simulink model "aa_IOT"  (R2024b)
settings: Solver=VariableStepAuto  StartTime=0.0  StopTime=0.05  RelTol=1e-3
undefined symbols (not defined in the file): Acid, Ion, Lead, Lithium, sigbuilder_block
libraries: spsBreakerLib x120, spsBatteryLib x82, spsSeriesRLCBranchLib x74, spsIdealSwitchLib x37, spsVoltageMeasurementLib x29, slpidlib x17, spsMosfetLib x17, spsPWMGeneratorDCDCLib x11, spsDiodeLib x10, spsIGBTLib x4, spsCurrentMeasurementLib x4, spsThreePhaseSeriesRLCLoadLib x2
(part 3 of 6)

== system aa_IOT/Subsystem11/Subsystem29 ==
  Battery : spsBatteryLib/Battery  BatType=Lithium-Ion  NomV=12  NomQ=10  SOC=95  Batt_Tr=30  PresetModel=on  MaxQ=10  MinV=9  FullV=13.9678  Dis_rate=4.3478  R=0.012  Normal_OP=9.0435  expZone="[12.9646     0.491304]"
  Breaker{,1..3} (4 alike) : spsBreakerLib/Breaker  InitialState=0  SwitchingTimes="[1/60  5/60]"  External=on  BreakerResistance=0.01  SnubberResistance=1e6  SnubberCapacitance=inf  Measurements=None  MoreParameters=on  NoBreakLoop=off
  Bus Selector : BusSelector  OutputSignals=SOC (%),Current (A),Voltage (V)
  Scope : Scope  NumInputPorts=3
  Series RLC Branch : spsSeriesRLCBranchLib/Series RLC Branch  LConnTagsString=__new0  RConnTagsString=__new0  BranchType=R  Resistance=1  Inductance=1e-3  SetiL0=off  InitialCurrent=0  Capacitance=1e-6  Setx0=off  InitialVoltage=0  Measurements=None
  + : PMIOPort  Side=Right
  - : PMIOPort  Port=2  Side=Right
  tag scope: s22=global
  wires:
  Battery/1 -> Bus Selector/1
  [c22] -> Breaker3/1, Breaker/1
  Bus Selector/2 -> Scope/2  "<Current (A)>"
  [d22] -> Breaker1/1, Breaker2/1
  Bus Selector/3 -> Scope/3  "<Voltage (V)>"
  Bus Selector/1 -> [s22], Scope/1  "<SOC (%)>"
  connections:
  Breaker2/LConn1 -- Breaker3/RConn1 -- Battery/LConn2
  Breaker1/LConn1 -- Battery/LConn1 -- Breaker/RConn1
  +/RConn1 -- Breaker/LConn1
  Series RLC Branch/LConn1 -- Breaker2/RConn1
  Series RLC Branch/RConn1 -- Breaker1/RConn1
  -/RConn1 -- Breaker3/LConn1

== system aa_IOT/Subsystem11/Subsystem3 ==
  Battery : spsBatteryLib/Battery  BatType=Lithium-Ion  NomV=12  NomQ=10  SOC=95  Batt_Tr=30  PresetModel=on  MaxQ=10  MinV=9  FullV=13.9678  Dis_rate=4.3478  R=0.012  Normal_OP=9.0435  expZone="[12.9646     0.491304]"
  Breaker{,1..3} (4 alike) : spsBreakerLib/Breaker  InitialState=0  SwitchingTimes="[1/60  5/60]"  External=on  BreakerResistance=0.01  SnubberResistance=1e6  SnubberCapacitance=inf  Measurements=None  MoreParameters=on  NoBreakLoop=off
  Bus Selector : BusSelector  OutputSignals=SOC (%),Current (A),Voltage (V)
  Scope : Scope  NumInputPorts=3
  Series RLC Branch : spsSeriesRLCBranchLib/Series RLC Branch  LConnTagsString=__new0  RConnTagsString=__new0  BranchType=R  Resistance=1  Inductance=1e-3  SetiL0=off  InitialCurrent=0  Capacitance=1e-6  Setx0=off  InitialVoltage=0  Measurements=None
  + : PMIOPort  Side=Right
  - : PMIOPort  Port=2  Side=Right
  tag scope: s4=global
  wires:
  Battery/1 -> Bus Selector/1
  [c4] -> Breaker3/1, Breaker/1
  Bus Selector/2 -> Scope/2  "<Current (A)>"
  [d4] -> Breaker1/1, Breaker2/1
  Bus Selector/3 -> Scope/3  "<Voltage (V)>"
  Bus Selector/1 -> [s4], Scope/1  "<SOC (%)>"
  connections:
  Breaker2/LConn1 -- Breaker3/RConn1 -- Battery/LConn2
  Breaker1/LConn1 -- Battery/LConn1 -- Breaker/RConn1
  +/RConn1 -- Breaker/LConn1
  Series RLC Branch/LConn1 -- Breaker2/RConn1
  Series RLC Branch/RConn1 -- Breaker1/RConn1
  -/RConn1 -- Breaker3/LConn1

== system aa_IOT/Subsystem11/Subsystem4 ==
  Battery : spsBatteryLib/Battery  BatType=Lithium-Ion  NomV=12  NomQ=10  SOC=95  Batt_Tr=30  PresetModel=on  MaxQ=10  MinV=9  FullV=13.9678  Dis_rate=4.3478  R=0.012  Normal_OP=9.0435  expZone="[12.9646     0.491304]"
  Breaker{,1..3} (4 alike) : spsBreakerLib/Breaker  InitialState=0  SwitchingTimes="[1/60  5/60]"  External=on  BreakerResistance=0.01  SnubberResistance=1e6  SnubberCapacitance=inf  Measurements=None  MoreParameters=on  NoBreakLoop=off
  Bus Selector : BusSelector  OutputSignals=SOC (%),Current (A),Voltage (V)
  Scope : Scope  NumInputPorts=3
  Series RLC Branch : spsSeriesRLCBranchLib/Series RLC Branch  LConnTagsString=__new0  RConnTagsString=__new0  BranchType=R  Resistance=1  Inductance=1e-3  SetiL0=off  InitialCurrent=0  Capacitance=1e-6  Setx0=off  InitialVoltage=0  Measurements=None
  + : PMIOPort  Side=Right
  - : PMIOPort  Port=2  Side=Right
  tag scope: s3=global
  wires:
  Battery/1 -> Bus Selector/1
  [c3] -> Breaker3/1, Breaker/1
  Bus Selector/2 -> Scope/2  "<Current (A)>"
  [d3] -> Breaker1/1, Breaker2/1
  Bus Selector/3 -> Scope/3  "<Voltage (V)>"
  Bus Selector/1 -> [s3], Scope/1  "<SOC (%)>"
  connections:
  Breaker2/LConn1 -- Breaker3/RConn1 -- Battery/LConn2
  Breaker1/LConn1 -- Battery/LConn1 -- Breaker/RConn1
  +/RConn1 -- Breaker/LConn1
  Series RLC Branch/LConn1 -- Breaker2/RConn1
  Series RLC Branch/RConn1 -- Breaker1/RConn1
  -/RConn1 -- Breaker3/LConn1

== system aa_IOT/Subsystem11/Subsystem5 ==
  Battery : spsBatteryLib/Battery  BatType=Lithium-Ion  NomV=12  NomQ=10  SOC=95  Batt_Tr=30  PresetModel=on  MaxQ=10  MinV=9  FullV=13.9678  Dis_rate=4.3478  R=0.012  Normal_OP=9.0435  expZone="[12.9646     0.491304]"
  Breaker{,1..3} (4 alike) : spsBreakerLib/Breaker  InitialState=0  SwitchingTimes="[1/60  5/60]"  External=on  BreakerResistance=0.01  SnubberResistance=1e6  SnubberCapacitance=inf  Measurements=None  MoreParameters=on  NoBreakLoop=off
  Bus Selector : BusSelector  OutputSignals=SOC (%),Current (A),Voltage (V)
  Scope : Scope  NumInputPorts=3
  Series RLC Branch : spsSeriesRLCBranchLib/Series RLC Branch  LConnTagsString=__new0  RConnTagsString=__new0  BranchType=R  Resistance=1  Inductance=1e-3  SetiL0=off  InitialCurrent=0  Capacitance=1e-6  Setx0=off  InitialVoltage=0  Measurements=None
  + : PMIOPort  Side=Right
  - : PMIOPort  Port=2  Side=Right
  tag scope: s2=global
  wires:
  Battery/1 -> Bus Selector/1
  [c2] -> Breaker3/1, Breaker/1
  Bus Selector/2 -> Scope/2  "<Current (A)>"
  [d2] -> Breaker1/1, Breaker2/1
  Bus Selector/3 -> Scope/3  "<Voltage (V)>"
  Bus Selector/1 -> [s2], Scope/1  "<SOC (%)>"
  connections:
  Breaker2/LConn1 -- Breaker3/RConn1 -- Battery/LConn2
  Breaker1/LConn1 -- Battery/LConn1 -- Breaker/RConn1
  +/RConn1 -- Breaker/LConn1
  Series RLC Branch/LConn1 -- Breaker2/RConn1
  Series RLC Branch/RConn1 -- Breaker1/RConn1
  -/RConn1 -- Breaker3/LConn1

== system aa_IOT/Subsystem11/Subsystem6 ==
  Battery : spsBatteryLib/Battery  BatType=Lithium-Ion  NomV=12  NomQ=10  SOC=95  Batt_Tr=30  PresetModel=on  MaxQ=10  MinV=9  FullV=13.9678  Dis_rate=4.3478  R=0.012  Normal_OP=9.0435  expZone="[12.9646     0.491304]"
  Breaker{,1..3} (4 alike) : spsBreakerLib/Breaker  InitialState=0  SwitchingTimes="[1/60  5/60]"  External=on  BreakerResistance=0.01  SnubberResistance=1e6  SnubberCapacitance=inf  Measurements=None  MoreParameters=on  NoBreakLoop=off
  Bus Selector : BusSelector  OutputSignals=SOC (%),Current (A),Voltage (V)
  Scope : Scope  NumInputPorts=3
  Series RLC Branch : spsSeriesRLCBranchLib/Series RLC Branch  LConnTagsString=__new0  RConnTagsString=__new0  BranchType=R  Resistance=1  Inductance=1e-3  SetiL0=off  InitialCurrent=0  Capacitance=1e-6  Setx0=off  InitialVoltage=0  Measurements=None
  + : PMIOPort  Side=Right
  - : PMIOPort  Port=2  Side=Right
  tag scope: s15=global
  wires:
  Battery/1 -> Bus Selector/1
  [c15] -> Breaker3/1, Breaker/1
  Bus Selector/2 -> Scope/2  "<Current (A)>"
  [d15] -> Breaker1/1, Breaker2/1
  Bus Selector/3 -> Scope/3  "<Voltage (V)>"
  Bus Selector/1 -> [s15], Scope/1  "<SOC (%)>"
  connections:
  Breaker2/LConn1 -- Breaker3/RConn1 -- Battery/LConn2
  Breaker1/LConn1 -- Battery/LConn1 -- Breaker/RConn1
  +/RConn1 -- Breaker/LConn1
  Series RLC Branch/LConn1 -- Breaker2/RConn1
  Series RLC Branch/RConn1 -- Breaker1/RConn1
  -/RConn1 -- Breaker3/LConn1

== system aa_IOT/Subsystem11/Subsystem7 ==
  Battery : spsBatteryLib/Battery  BatType=Lithium-Ion  NomV=12  NomQ=10  SOC=95  Batt_Tr=30  PresetModel=on  MaxQ=10  MinV=9  FullV=13.9678  Dis_rate=4.3478  R=0.012  Normal_OP=9.0435  expZone="[12.9646     0.491304]"
  Breaker{,1..3} (4 alike) : spsBreakerLib/Breaker  InitialState=0  SwitchingTimes="[1/60  5/60]"  External=on  BreakerResistance=0.01  SnubberResistance=1e6  SnubberCapacitance=inf  Measurements=None  MoreParameters=on  NoBreakLoop=off
  Bus Selector : BusSelector  OutputSignals=SOC (%),Current (A),Voltage (V)
  Scope : Scope  NumInputPorts=3
  Series RLC Branch : spsSeriesRLCBranchLib/Series RLC Branch  LConnTagsString=__new0  RConnTagsString=__new0  BranchType=R  Resistance=1  Inductance=1e-3  SetiL0=off  InitialCurrent=0  Capacitance=1e-6  Setx0=off  InitialVoltage=0  Measurements=None
  + : PMIOPort  Side=Right
  - : PMIOPort  Port=2  Side=Right
  tag scope: s11=global
  wires:
  Battery/1 -> Bus Selector/1
  [c11] -> Breaker3/1, Breaker/1
  Bus Selector/2 -> Scope/2  "<Current (A)>"
  [d11] -> Breaker1/1, Breaker2/1
  Bus Selector/3 -> Scope/3  "<Voltage (V)>"
  Bus Selector/1 -> [s11], Scope/1  "<SOC (%)>"
  connections:
  Breaker2/LConn1 -- Breaker3/RConn1 -- Battery/LConn2
  Breaker1/LConn1 -- Battery/LConn1 -- Breaker/RConn1
  +/RConn1 -- Breaker/LConn1
  Series RLC Branch/LConn1 -- Breaker2/RConn1
  Series RLC Branch/RConn1 -- Breaker1/RConn1
  -/RConn1 -- Breaker3/LConn1

== system aa_IOT/Subsystem11/Subsystem8 ==
  Battery : spsBatteryLib/Battery  BatType=Lithium-Ion  NomV=12  NomQ=10  SOC=95  Batt_Tr=30  PresetModel=on  MaxQ=10  MinV=9  FullV=13.9678  Dis_rate=4.3478  R=0.012  Normal_OP=9.0435  expZone="[12.9646     0.491304]"
  Breaker{,1..3} (4 alike) : spsBreakerLib/Breaker  InitialState=0  SwitchingTimes="[1/60  5/60]"  External=on  BreakerResistance=0.01  SnubberResistance=1e6  SnubberCapacitance=inf  Measurements=None  MoreParameters=on  NoBreakLoop=off
  Bus Selector : BusSelector  OutputSignals=SOC (%),Current (A),Voltage (V)
  Scope : Scope  NumInputPorts=3
  Series RLC Branch : spsSeriesRLCBranchLib/Series RLC Branch  LConnTagsString=__new0  RConnTagsString=__new0  BranchType=R  Resistance=1  Inductance=1e-3  SetiL0=off  InitialCurrent=0  Capacitance=1e-6  Setx0=off  InitialVoltage=0  Measurements=None
  + : PMIOPort  Side=Right
  - : PMIOPort  Port=2  Side=Right
  tag scope: s19=global
  wires:
  Battery/1 -> Bus Selector/1
  [c19] -> Breaker3/1, Breaker/1
  Bus Selector/2 -> Scope/2  "<Current (A)>"
  [d19] -> Breaker1/1, Breaker2/1
  Bus Selector/3 -> Scope/3  "<Voltage (V)>"
  Bus Selector/1 -> [s19], Scope/1  "<SOC (%)>"
  connections:
  Breaker2/LConn1 -- Breaker3/RConn1 -- Battery/LConn2
  Breaker1/LConn1 -- Battery/LConn1 -- Breaker/RConn1
  +/RConn1 -- Breaker/LConn1
  Series RLC Branch/LConn1 -- Breaker2/RConn1
  Series RLC Branch/RConn1 -- Breaker1/RConn1
  -/RConn1 -- Breaker3/LConn1

== system aa_IOT/Subsystem11/Subsystem9 ==
  Battery : spsBatteryLib/Battery  BatType=Lithium-Ion  NomV=12  NomQ=10  SOC=95  Batt_Tr=30  PresetModel=on  MaxQ=10  MinV=9  FullV=13.9678  Dis_rate=4.3478  R=0.012  Normal_OP=9.0435  expZone="[12.9646     0.491304]"
  Breaker{,1..3} (4 alike) : spsBreakerLib/Breaker  InitialState=0  SwitchingTimes="[1/60  5/60]"  External=on  BreakerResistance=0.01  SnubberResistance=1e6  SnubberCapacitance=inf  Measurements=None  MoreParameters=on  NoBreakLoop=off
  Bus Selector : BusSelector  OutputSignals=SOC (%),Current (A),Voltage (V)
  Scope : Scope  NumInputPorts=3
  Series RLC Branch : spsSeriesRLCBranchLib/Series RLC Branch  LConnTagsString=__new0  RConnTagsString=__new0  BranchType=R  Resistance=1  Inductance=1e-3  SetiL0=off  InitialCurrent=0  Capacitance=1e-6  Setx0=off  InitialVoltage=0  Measurements=None
  + : PMIOPort  Side=Right
  - : PMIOPort  Port=2  Side=Right
  tag scope: s20=global
  wires:
  Battery/1 -> Bus Selector/1
  [c20] -> Breaker3/1, Breaker/1
  Bus Selector/2 -> Scope/2  "<Current (A)>"
  [d20] -> Breaker1/1, Breaker2/1
  Bus Selector/3 -> Scope/3  "<Voltage (V)>"
  Bus Selector/1 -> [s20], Scope/1  "<SOC (%)>"
  connections:
  Breaker2/LConn1 -- Breaker3/RConn1 -- Battery/LConn2
  Breaker1/LConn1 -- Battery/LConn1 -- Breaker/RConn1
  +/RConn1 -- Breaker/LConn1
  Series RLC Branch/LConn1 -- Breaker2/RConn1
  Series RLC Branch/RConn1 -- Breaker1/RConn1
  -/RConn1 -- Breaker3/LConn1

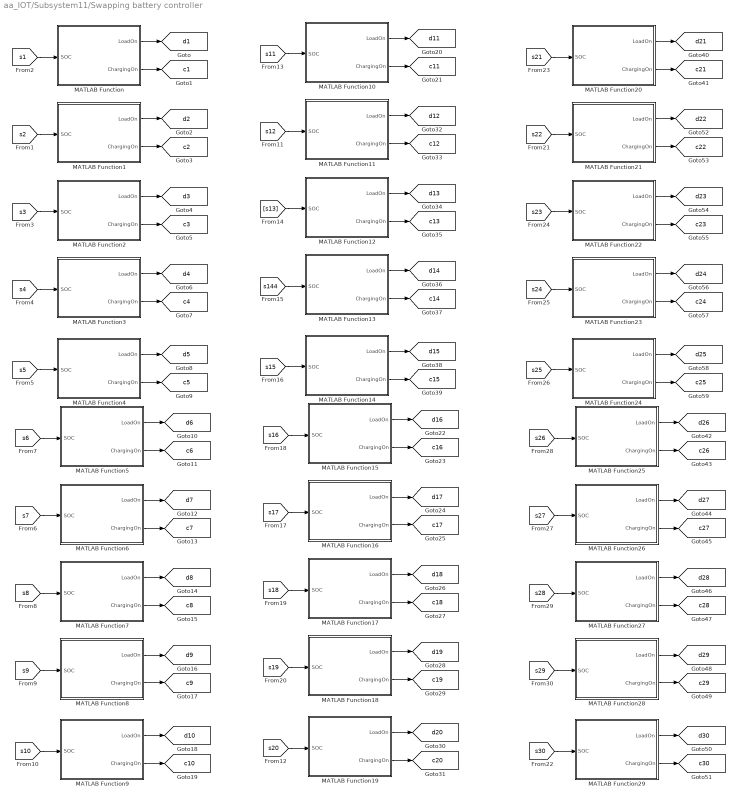
== system aa_IOT/Subsystem11/Swapping battery controller ==
  MATLAB Function : MATLAB Function  TreatAsAtomicUnit=on
  MATLAB Function1 : MATLAB Function  TreatAsAtomicUnit=on
  MATLAB Function10 : MATLAB Function  TreatAsAtomicUnit=on
  MATLAB Function11 : MATLAB Function  TreatAsAtomicUnit=on
  MATLAB Function12 : MATLAB Function  TreatAsAtomicUnit=on
  MATLAB Function13 : MATLAB Function  TreatAsAtomicUnit=on
  MATLAB Function14 : MATLAB Function  TreatAsAtomicUnit=on
  MATLAB Function15 : MATLAB Function  TreatAsAtomicUnit=on
  MATLAB Function16 : MATLAB Function  TreatAsAtomicUnit=on
  MATLAB Function17 : MATLAB Function  TreatAsAtomicUnit=on
  MATLAB Function18 : MATLAB Function  TreatAsAtomicUnit=on
  MATLAB Function19 : MATLAB Function  TreatAsAtomicUnit=on
  MATLAB Function2 : MATLAB Function  TreatAsAtomicUnit=on
  MATLAB Function20 : MATLAB Function  TreatAsAtomicUnit=on
  MATLAB Function21 : MATLAB Function  TreatAsAtomicUnit=on
  MATLAB Function22 : MATLAB Function  TreatAsAtomicUnit=on
  MATLAB Function23 : MATLAB Function  TreatAsAtomicUnit=on
  MATLAB Function24 : MATLAB Function  TreatAsAtomicUnit=on
  MATLAB Function25 : MATLAB Function  TreatAsAtomicUnit=on
  MATLAB Function26 : MATLAB Function  TreatAsAtomicUnit=on
  MATLAB Function27 : MATLAB Function  TreatAsAtomicUnit=on
  MATLAB Function28 : MATLAB Function  TreatAsAtomicUnit=on
  MATLAB Function29 : MATLAB Function  TreatAsAtomicUnit=on
  MATLAB Function3 : MATLAB Function  TreatAsAtomicUnit=on
  MATLAB Function4 : MATLAB Function  TreatAsAtomicUnit=on
  MATLAB Function5 : MATLAB Function  TreatAsAtomicUnit=on
  MATLAB Function6 : MATLAB Function  TreatAsAtomicUnit=on
  MATLAB Function7 : MATLAB Function  TreatAsAtomicUnit=on
  MATLAB Function8 : MATLAB Function  TreatAsAtomicUnit=on
  MATLAB Function9 : MATLAB Function  TreatAsAtomicUnit=on
  tag scope: c10=global, c11=global, c12=global, c13=global, c14=global, c15=global, c16=global, c17=global, c18=global, c19=global, c1=global, c20=global, c21=global, c22=global, c23=global, c24=global, c25=global, c26=global, c27=global, c28=global, c29=global, c2=global, c30=global, c3=global, c4=global, c5=global, c6=global, c7=global, c8=global, c9=global, d10=global, d11=global, d12=global, d13=global, d14=global, d15=global, d16=global, d17=global, d18=global, d19=global, d1=global, d20=global, d21=global, d22=global, d23=global, d24=global, d25=global, d26=global, d27=global, d28=global, d29=global, d2=global, d30=global, d3=global, d4=global, d5=global, d6=global, d7=global, d8=global, d9=global
  wires:
  MATLAB Function10/1(LoadOn) -> [d11]
  MATLAB Function1/2(ChargingOn) -> [c2]
  [s20] -> MATLAB Function19/1(SOC)
  [s22] -> MATLAB Function21/1(SOC)
  MATLAB Function5/1(LoadOn) -> [d6]
  [s16] -> MATLAB Function15/1(SOC)
  [s5] -> MATLAB Function4/1(SOC)
  MATLAB Function/2(ChargingOn) -> [c1]
  MATLAB Function2/2(ChargingOn) -> [c3]
  MATLAB Function26/1(LoadOn) -> [d27]
  [s21] -> MATLAB Function20/1(SOC)
  MATLAB Function18/1(LoadOn) -> [d19]
  MATLAB Function7/2(ChargingOn) -> [c8]
  MATLAB Function12/2(ChargingOn) -> [c13]
  MATLAB Function28/1(LoadOn) -> [d29]
  MATLAB Function4/2(ChargingOn) -> [c5]
  MATLAB Function25/2(ChargingOn) -> [c26]
  [s1] -> MATLAB Function/1(SOC)
  MATLAB Function11/2(ChargingOn) -> [c12]
  MATLAB Function/1(LoadOn) -> [d1]
  MATLAB Function16/1(LoadOn) -> [d17]
  MATLAB Function10/2(ChargingOn) -> [c11]
  [s15] -> MATLAB Function14/1(SOC)
  [s12] -> MATLAB Function11/1(SOC)
  [s3] -> MATLAB Function2/1(SOC)
  MATLAB Function2/1(LoadOn) -> [d3]
  MATLAB Function17/1(LoadOn) -> [d18]
  MATLAB Function13/2(ChargingOn) -> [c14]
  MATLAB Function4/1(LoadOn) -> [d5]
  MATLAB Function14/2(ChargingOn) -> [c15]
  MATLAB Function3/1(LoadOn) -> [d4]
  MATLAB Function6/2(ChargingOn) -> [c7]
  [s7] -> MATLAB Function6/1(SOC)
  MATLAB Function15/1(LoadOn) -> [d16]
  MATLAB Function26/2(ChargingOn) -> [c27]
  [s8] -> MATLAB Function7/1(SOC)
  MATLAB Function6/1(LoadOn) -> [d7]
  MATLAB Function13/1(LoadOn) -> [d14]
  MATLAB Function16/2(ChargingOn) -> [c17]
  MATLAB Function18/2(ChargingOn) -> [c19]
  MATLAB Function5/2(ChargingOn) -> [c6]
  [s6] -> MATLAB Function5/1(SOC)
  [s18] -> MATLAB Function17/1(SOC)
  [s13] -> MATLAB Function12/1(SOC)
  MATLAB Function19/2(ChargingOn) -> [c20]
  MATLAB Function22/1(LoadOn) -> [d23]
  [s27] -> MATLAB Function26/1(SOC)
  MATLAB Function19/1(LoadOn) -> [d20]
  [s26] -> MATLAB Function25/1(SOC)
  [s29] -> MATLAB Function28/1(SOC)
  MATLAB Function8/2(ChargingOn) -> [c9]
  [s17] -> MATLAB Function16/1(SOC)
  MATLAB Function17/2(ChargingOn) -> [c18]
  [s19] -> MATLAB Function18/1(SOC)
  MATLAB Function3/2(ChargingOn) -> [c4]
  MATLAB Function11/1(LoadOn) -> [d12]
  [s11] -> MATLAB Function10/1(SOC)
  MATLAB Function8/1(LoadOn) -> [d9]
  [s2] -> MATLAB Function1/1(SOC)
  MATLAB Function12/1(LoadOn) -> [d13]
  [s10] -> MATLAB Function9/1(SOC)
  MATLAB Function14/1(LoadOn) -> [d15]
  [s144] -> MATLAB Function13/1(SOC)
  MATLAB Function1/1(LoadOn) -> [d2]
  [s4] -> MATLAB Function3/1(SOC)
  MATLAB Function15/2(ChargingOn) -> [c16]
  MATLAB Function7/1(LoadOn) -> [d8]
  [s9] -> MATLAB Function8/1(SOC)
  MATLAB Function9/1(LoadOn) -> [d10]
  MATLAB Function9/2(ChargingOn) -> [c10]
  MATLAB Function29/2(ChargingOn) -> [c30]
  MATLAB Function29/1(LoadOn) -> [d30]
  MATLAB Function27/2(ChargingOn) -> [c28]
  MATLAB Function25/1(LoadOn) -> [d26]
  [s28] -> MATLAB Function27/1(SOC)
  [s30] -> MATLAB Function29/1(SOC)
  MATLAB Function28/2(ChargingOn) -> [c29]
  MATLAB Function23/1(LoadOn) -> [d24]
  [s24] -> MATLAB Function23/1(SOC)
  MATLAB Function23/2(ChargingOn) -> [c24]
  MATLAB Function21/1(LoadOn) -> [d22]
  MATLAB Function27/1(LoadOn) -> [d28]
  MATLAB Function24/1(LoadOn) -> [d25]
  MATLAB Function22/2(ChargingOn) -> [c23]
  [s23] -> MATLAB Function22/1(SOC)
  MATLAB Function24/2(ChargingOn) -> [c25]
  [s25] -> MATLAB Function24/1(SOC)
  MATLAB Function20/2(ChargingOn) -> [c21]
  MATLAB Function21/2(ChargingOn) -> [c22]
  MATLAB Function20/1(LoadOn) -> [d21]

== system aa_IOT/Subsystem2/Control ==
  Add : Sum  Inputs=+-
  Add1 : Sum  Inputs=+-
  Constant : Constant  Value=25.99
  Gain : Gain  Gain=-1
  NOT : Logic  Operator=NOT  IconShape=distinctive  AllPortsSameDT=off  OutDataTypeStr=boolean
  PID Controller : slpidlib/PID Controller  Controller=PI  Form=Parallel  TimeDomain=Continuous-time  UseExternalTs=off  SampleTime=-1  IntegratorMethod=Forward Euler  FilterMethod=Forward Euler  ControllerParametersSource=internal  P=0.005  I=10  UseKiTs=off  D=0  UseExternalDerivativeSource=off  N=100  UseFilter=on  TunerSelectOption=Transfer Function Based (PID Tuner App)  InitialConditionSource=internal  InitialConditionForIntegrator=0.54  InitialConditionForFilter=0  DifferentiatorICPrevScaledInput=0  ExternalReset=none  TrackingMode=off  Kt=1  LimitOutput=on  SatLimitsSource=internal  UpperSaturationLimit=0.975  LowerSaturationLimit=0  LinearizeAsGain=on  AntiWindupMode=none  Kb=1  LimitIntegrator=off  UpperIntegratorSaturationLimit=inf  LowerIntegratorSaturationLimit=-inf  POutMin=[]  POutMax=[]  IOutMin=[]  IOutMax=[]  DOutMin=[]  DOutMax=[]  NOutMin=[]  NOutMax=[]  SumOutMin=[]  SumOutMax=[]  SaturationOutMin=[]  SaturationOutMax=[]  PParamMin=[]  PParamMax=[]  IParamMin=[]  IParamMax=[]  DParamMin=[]  DParamMax=[]  NParamMin=[]  NParamMax=[]  KbParamMin=[]  KbParamMax=[]  KtParamMin=[]  KtParamMax=[]  KbOutMin=[]  KbOutMax=[]  KtOutMin=[]  KtOutMax=[]  IntegratorOutMin=[]  IntegratorOutMax=[]  FilterOutMin=[]  FilterOutMax=[]  SumI1OutMin=[]  SumI1OutMax=[]  SumI2OutMin=[]  SumI2OutMax=[]  SumI3OutMin=[]  SumI3OutMax=[]  SumI4OutMin=[]  SumI4OutMax=[]  SumDOutMin=[]  SumDOutMax=[]  DifferentiatorOutMin=[]  DifferentiatorOutMax=[]  FilterDiffOutCoefMin=[]  FilterDiffOutCoefMax=[]  ReciprocalOutMin=[]  ReciprocalOutMax=[]  SumDenOutMin=[]  SumDenOutMax=[]  SumNumOutMin=[]  SumNumOutMax=[]  DivideOutMin=[]  DivideOutMax=[]  UdiffTsProdOutMin=[]  UdiffTsProdOutMax=[]  NTsProdOutMin=[]  NTsProdOutMax=[]  UintegralTsProdOutMin=[]  UintegralTsProdOutMax=[]  UngainTsProdOutMin=[]  UngainTsProdOutMax=[]  ClampingZeroOutDataTypeStr=Inherit: Inherit via back propagation  ClampingZeroOutMin=[]  ClampingZeroOutMax=[]  FilterDenConstantOutDataTypeStr=Inherit: Inherit via back propagation  FilterDenConstantOutMin=[]  FilterDenConstantOutMax=[]  PCopyOutDataTypeStr=Inherit: Inherit via back propagation  PCopyOutMin=[]  PCopyOutMax=[]  NCopyOutDataTypeStr=Inherit: Inherit via back propagation  NCopyOutMin=[]  NCopyOutMax=[]  IntegratorContinuousStateAttributes=''  IntegratorStateMustResolveToSignalObject=off  IntegratorRTWStateStorageClass=Auto  FilterContinuousStateAttributes=''  FilterStateMustResolveToSignalObject=off  FilterRTWStateStorageClass=Auto  ParallelPVariant=InternalParameters  IdealPVariant=Disabled  IVariant=InternalParameters  DVariant=Disabled  IntegratorVariant=Continuous  SatVariant=Enabled  AWVariant=Passthrough  PCopyVariant=Disabled  TRVariant=Disabled  FdbkBlocksVariant=Forward  IdealPFdbkVariant=Disabled  SatFdbkVariant=Disabled  DerivativeFilterVariant=Disabled  NVariant=Disabled  NCopyVariant=Disabled_SignalSpec  FilterICVariant=Disabled  IntegratorICVariant=InternalICs  ExternalResetVariant=Disabled  TRSumVariant=Passthrough  SumFdbkVariant=Disabled  SumVariant=Sum_PI  TsampFilterVariant=InternalTs  TsampNgainVariant=Passthrough  TsampIntegralVariant=Disabled_SignalSpec  ExternalSaturationOutDataTypeStr=Inherit: Same as second input  DerivativeSourceVariant=Disabled  PreIntVariant=InternalPreInt
  PID Controller1 : slpidlib/PID Controller  Controller=PI  Form=Parallel  TimeDomain=Continuous-time  UseExternalTs=off  SampleTime=-1  IntegratorMethod=Forward Euler  FilterMethod=Forward Euler  ControllerParametersSource=internal  P=40  I=2000  UseKiTs=off  D=0  UseExternalDerivativeSource=off  N=100  UseFilter=on  TunerSelectOption=Transfer Function Based (PID Tuner App)  InitialConditionSource=internal  InitialConditionForIntegrator=0.54  InitialConditionForFilter=0  DifferentiatorICPrevScaledInput=0  ExternalReset=none  TrackingMode=off  Kt=1  LimitOutput=on  SatLimitsSource=internal  UpperSaturationLimit=17.39  LowerSaturationLimit=0  LinearizeAsGain=on  AntiWindupMode=none  Kb=1  LimitIntegrator=off  UpperIntegratorSaturationLimit=inf  LowerIntegratorSaturationLimit=-inf  POutMin=[]  POutMax=[]  IOutMin=[]  IOutMax=[]  DOutMin=[]  DOutMax=[]  NOutMin=[]  NOutMax=[]  SumOutMin=[]  SumOutMax=[]  SaturationOutMin=[]  SaturationOutMax=[]  PParamMin=[]  PParamMax=[]  IParamMin=[]  IParamMax=[]  DParamMin=[]  DParamMax=[]  NParamMin=[]  NParamMax=[]  KbParamMin=[]  KbParamMax=[]  KtParamMin=[]  KtParamMax=[]  KbOutMin=[]  KbOutMax=[]  KtOutMin=[]  KtOutMax=[]  IntegratorOutMin=[]  IntegratorOutMax=[]  FilterOutMin=[]  FilterOutMax=[]  SumI1OutMin=[]  SumI1OutMax=[]  SumI2OutMin=[]  SumI2OutMax=[]  SumI3OutMin=[]  SumI3OutMax=[]  SumI4OutMin=[]  SumI4OutMax=[]  SumDOutMin=[]  SumDOutMax=[]  DifferentiatorOutMin=[]  DifferentiatorOutMax=[]  FilterDiffOutCoefMin=[]  FilterDiffOutCoefMax=[]  ReciprocalOutMin=[]  ReciprocalOutMax=[]  SumDenOutMin=[]  SumDenOutMax=[]  SumNumOutMin=[]  SumNumOutMax=[]  DivideOutMin=[]  DivideOutMax=[]  UdiffTsProdOutMin=[]  UdiffTsProdOutMax=[]  NTsProdOutMin=[]  NTsProdOutMax=[]  UintegralTsProdOutMin=[]  UintegralTsProdOutMax=[]  UngainTsProdOutMin=[]  UngainTsProdOutMax=[]  ClampingZeroOutDataTypeStr=Inherit: Inherit via back propagation  ClampingZeroOutMin=[]  ClampingZeroOutMax=[]  FilterDenConstantOutDataTypeStr=Inherit: Inherit via back propagation  FilterDenConstantOutMin=[]  FilterDenConstantOutMax=[]  PCopyOutDataTypeStr=Inherit: Inherit via back propagation  PCopyOutMin=[]  PCopyOutMax=[]  NCopyOutDataTypeStr=Inherit: Inherit via back propagation  NCopyOutMin=[]  NCopyOutMax=[]  IntegratorContinuousStateAttributes=''  IntegratorStateMustResolveToSignalObject=off  IntegratorRTWStateStorageClass=Auto  FilterContinuousStateAttributes=''  FilterStateMustResolveToSignalObject=off  FilterRTWStateStorageClass=Auto  ParallelPVariant=InternalParameters  IdealPVariant=Disabled  IVariant=InternalParameters  DVariant=Disabled  IntegratorVariant=Continuous  SatVariant=Enabled  AWVariant=Passthrough  PCopyVariant=Disabled  TRVariant=Disabled  FdbkBlocksVariant=Forward  IdealPFdbkVariant=Disabled  SatFdbkVariant=Disabled  DerivativeFilterVariant=Disabled  NVariant=Disabled  NCopyVariant=Disabled_SignalSpec  FilterICVariant=Disabled  IntegratorICVariant=InternalICs  ExternalResetVariant=Disabled  TRSumVariant=Passthrough  SumFdbkVariant=Disabled  SumVariant=Sum_PI  TsampFilterVariant=InternalTs  TsampNgainVariant=Passthrough  TsampIntegralVariant=Disabled_SignalSpec  ExternalSaturationOutDataTypeStr=Inherit: Same as second input  DerivativeSourceVariant=Disabled  PreIntVariant=InternalPreInt
  PWM Generator (DC-DC) : spsPWMGeneratorDCDCLib/PWM Generator (DC-DC)  Fsw=10e3  Ts=5e-6
  tag scope: Mosfet_333=global, Mosfet_33=global
  wires:
  Add/1 -> PID Controller/1
  PWM Generator (DC-DC)/1 -> NOT/1, [Mosfet_33]
  PID Controller/1 -> PWM Generator (DC-DC)/1
  NOT/1 -> [Mosfet_333]
  [Ref_Current] -> Add/2
  [Current] -> Add/1
  PID Controller1/1 -> Gain/1
  Gain/1 -> [Ref_Current]
  Add1/1 -> PID Controller1/1
  Constant/1 -> Add1/1
  [Voltage] -> Add1/2

== system aa_IOT/Subsystem3/Control ==
  Add : Sum  Inputs=+-
  Add1 : Sum  Inputs=+-
  Constant : Constant  Value=25.99
  Gain : Gain  Gain=-1
  NOT : Logic  Operator=NOT  IconShape=distinctive  AllPortsSameDT=off  OutDataTypeStr=boolean
  PID Controller : slpidlib/PID Controller  Controller=PI  Form=Parallel  TimeDomain=Continuous-time  UseExternalTs=off  SampleTime=-1  IntegratorMethod=Forward Euler  FilterMethod=Forward Euler  ControllerParametersSource=internal  P=0.005  I=10  UseKiTs=off  D=0  UseExternalDerivativeSource=off  N=100  UseFilter=on  TunerSelectOption=Transfer Function Based (PID Tuner App)  InitialConditionSource=internal  InitialConditionForIntegrator=0.54  InitialConditionForFilter=0  DifferentiatorICPrevScaledInput=0  ExternalReset=none  TrackingMode=off  Kt=1  LimitOutput=on  SatLimitsSource=internal  UpperSaturationLimit=0.975  LowerSaturationLimit=0  LinearizeAsGain=on  AntiWindupMode=none  Kb=1  LimitIntegrator=off  UpperIntegratorSaturationLimit=inf  LowerIntegratorSaturationLimit=-inf  POutMin=[]  POutMax=[]  IOutMin=[]  IOutMax=[]  DOutMin=[]  DOutMax=[]  NOutMin=[]  NOutMax=[]  SumOutMin=[]  SumOutMax=[]  SaturationOutMin=[]  SaturationOutMax=[]  PParamMin=[]  PParamMax=[]  IParamMin=[]  IParamMax=[]  DParamMin=[]  DParamMax=[]  NParamMin=[]  NParamMax=[]  KbParamMin=[]  KbParamMax=[]  KtParamMin=[]  KtParamMax=[]  KbOutMin=[]  KbOutMax=[]  KtOutMin=[]  KtOutMax=[]  IntegratorOutMin=[]  IntegratorOutMax=[]  FilterOutMin=[]  FilterOutMax=[]  SumI1OutMin=[]  SumI1OutMax=[]  SumI2OutMin=[]  SumI2OutMax=[]  SumI3OutMin=[]  SumI3OutMax=[]  SumI4OutMin=[]  SumI4OutMax=[]  SumDOutMin=[]  SumDOutMax=[]  DifferentiatorOutMin=[]  DifferentiatorOutMax=[]  FilterDiffOutCoefMin=[]  FilterDiffOutCoefMax=[]  ReciprocalOutMin=[]  ReciprocalOutMax=[]  SumDenOutMin=[]  SumDenOutMax=[]  SumNumOutMin=[]  SumNumOutMax=[]  DivideOutMin=[]  DivideOutMax=[]  UdiffTsProdOutMin=[]  UdiffTsProdOutMax=[]  NTsProdOutMin=[]  NTsProdOutMax=[]  UintegralTsProdOutMin=[]  UintegralTsProdOutMax=[]  UngainTsProdOutMin=[]  UngainTsProdOutMax=[]  ClampingZeroOutDataTypeStr=Inherit: Inherit via back propagation  ClampingZeroOutMin=[]  ClampingZeroOutMax=[]  FilterDenConstantOutDataTypeStr=Inherit: Inherit via back propagation  FilterDenConstantOutMin=[]  FilterDenConstantOutMax=[]  PCopyOutDataTypeStr=Inherit: Inherit via back propagation  PCopyOutMin=[]  PCopyOutMax=[]  NCopyOutDataTypeStr=Inherit: Inherit via back propagation  NCopyOutMin=[]  NCopyOutMax=[]  IntegratorContinuousStateAttributes=''  IntegratorStateMustResolveToSignalObject=off  IntegratorRTWStateStorageClass=Auto  FilterContinuousStateAttributes=''  FilterStateMustResolveToSignalObject=off  FilterRTWStateStorageClass=Auto  ParallelPVariant=InternalParameters  IdealPVariant=Disabled  IVariant=InternalParameters  DVariant=Disabled  IntegratorVariant=Continuous  SatVariant=Enabled  AWVariant=Passthrough  PCopyVariant=Disabled  TRVariant=Disabled  FdbkBlocksVariant=Forward  IdealPFdbkVariant=Disabled  SatFdbkVariant=Disabled  DerivativeFilterVariant=Disabled  NVariant=Disabled  NCopyVariant=Disabled_SignalSpec  FilterICVariant=Disabled  IntegratorICVariant=InternalICs  ExternalResetVariant=Disabled  TRSumVariant=Passthrough  SumFdbkVariant=Disabled  SumVariant=Sum_PI  TsampFilterVariant=InternalTs  TsampNgainVariant=Passthrough  TsampIntegralVariant=Disabled_SignalSpec  ExternalSaturationOutDataTypeStr=Inherit: Same as second input  DerivativeSourceVariant=Disabled  PreIntVariant=InternalPreInt
  PID Controller1 : slpidlib/PID Controller  Controller=PI  Form=Parallel  TimeDomain=Continuous-time  UseExternalTs=off  SampleTime=-1  IntegratorMethod=Forward Euler  FilterMethod=Forward Euler  ControllerParametersSource=internal  P=40  I=2000  UseKiTs=off  D=0  UseExternalDerivativeSource=off  N=100  UseFilter=on  TunerSelectOption=Transfer Function Based (PID Tuner App)  InitialConditionSource=internal  InitialConditionForIntegrator=0.54  InitialConditionForFilter=0  DifferentiatorICPrevScaledInput=0  ExternalReset=none  TrackingMode=off  Kt=1  LimitOutput=on  SatLimitsSource=internal  UpperSaturationLimit=17.39  LowerSaturationLimit=0  LinearizeAsGain=on  AntiWindupMode=none  Kb=1  LimitIntegrator=off  UpperIntegratorSaturationLimit=inf  LowerIntegratorSaturationLimit=-inf  POutMin=[]  POutMax=[]  IOutMin=[]  IOutMax=[]  DOutMin=[]  DOutMax=[]  NOutMin=[]  NOutMax=[]  SumOutMin=[]  SumOutMax=[]  SaturationOutMin=[]  SaturationOutMax=[]  PParamMin=[]  PParamMax=[]  IParamMin=[]  IParamMax=[]  DParamMin=[]  DParamMax=[]  NParamMin=[]  NParamMax=[]  KbParamMin=[]  KbParamMax=[]  KtParamMin=[]  KtParamMax=[]  KbOutMin=[]  KbOutMax=[]  KtOutMin=[]  KtOutMax=[]  IntegratorOutMin=[]  IntegratorOutMax=[]  FilterOutMin=[]  FilterOutMax=[]  SumI1OutMin=[]  SumI1OutMax=[]  SumI2OutMin=[]  SumI2OutMax=[]  SumI3OutMin=[]  SumI3OutMax=[]  SumI4OutMin=[]  SumI4OutMax=[]  SumDOutMin=[]  SumDOutMax=[]  DifferentiatorOutMin=[]  DifferentiatorOutMax=[]  FilterDiffOutCoefMin=[]  FilterDiffOutCoefMax=[]  ReciprocalOutMin=[]  ReciprocalOutMax=[]  SumDenOutMin=[]  SumDenOutMax=[]  SumNumOutMin=[]  SumNumOutMax=[]  DivideOutMin=[]  DivideOutMax=[]  UdiffTsProdOutMin=[]  UdiffTsProdOutMax=[]  NTsProdOutMin=[]  NTsProdOutMax=[]  UintegralTsProdOutMin=[]  UintegralTsProdOutMax=[]  UngainTsProdOutMin=[]  UngainTsProdOutMax=[]  ClampingZeroOutDataTypeStr=Inherit: Inherit via back propagation  ClampingZeroOutMin=[]  ClampingZeroOutMax=[]  FilterDenConstantOutDataTypeStr=Inherit: Inherit via back propagation  FilterDenConstantOutMin=[]  FilterDenConstantOutMax=[]  PCopyOutDataTypeStr=Inherit: Inherit via back propagation  PCopyOutMin=[]  PCopyOutMax=[]  NCopyOutDataTypeStr=Inherit: Inherit via back propagation  NCopyOutMin=[]  NCopyOutMax=[]  IntegratorContinuousStateAttributes=''  IntegratorStateMustResolveToSignalObject=off  IntegratorRTWStateStorageClass=Auto  FilterContinuousStateAttributes=''  FilterStateMustResolveToSignalObject=off  FilterRTWStateStorageClass=Auto  ParallelPVariant=InternalParameters  IdealPVariant=Disabled  IVariant=InternalParameters  DVariant=Disabled  IntegratorVariant=Continuous  SatVariant=Enabled  AWVariant=Passthrough  PCopyVariant=Disabled  TRVariant=Disabled  FdbkBlocksVariant=Forward  IdealPFdbkVariant=Disabled  SatFdbkVariant=Disabled  DerivativeFilterVariant=Disabled  NVariant=Disabled  NCopyVariant=Disabled_SignalSpec  FilterICVariant=Disabled  IntegratorICVariant=InternalICs  ExternalResetVariant=Disabled  TRSumVariant=Passthrough  SumFdbkVariant=Disabled  SumVariant=Sum_PI  TsampFilterVariant=InternalTs  TsampNgainVariant=Passthrough  TsampIntegralVariant=Disabled_SignalSpec  ExternalSaturationOutDataTypeStr=Inherit: Same as second input  DerivativeSourceVariant=Disabled  PreIntVariant=InternalPreInt
  PWM Generator (DC-DC) : spsPWMGeneratorDCDCLib/PWM Generator (DC-DC)  Fsw=10e3  Ts=5e-6
  tag scope: Mosfet_444=global, Mosfet_44=global
  wires:
  Add/1 -> PID Controller/1
  PWM Generator (DC-DC)/1 -> NOT/1, [Mosfet_44]
  PID Controller/1 -> PWM Generator (DC-DC)/1
  NOT/1 -> [Mosfet_444]
  [Ref_Current] -> Add/2
  [Current] -> Add/1
  PID Controller1/1 -> Gain/1
  Gain/1 -> [Ref_Current]
  Add1/1 -> PID Controller1/1
  Constant/1 -> Add1/1
  [Voltage] -> Add1/2

== system aa_IOT/Subsystem4/Subsystem ==
  Battery1 : spsBatteryLib/Battery  BatType=Lithium-Ion  NomV=3.6  NomQ=4  SOC=100  Batt_Tr=1  PresetModel=on  MaxQ=4  MinV=2.7  FullV=4.1904  Dis_rate=1.7391  R=0.009  Normal_OP=3.6174  expZone="[3.8894     0.19652]"
  Battery2 : spsBatteryLib/Battery  BatType=Lithium-Ion  NomV=3.6  NomQ=4  SOC=60  Batt_Tr=1  PresetModel=on  MaxQ=4  MinV=2.7  FullV=4.1904  Dis_rate=1.7391  R=0.009  Normal_OP=3.6174  expZone="[3.8894     0.19652]"
  Battery3 : spsBatteryLib/Battery  BatType=Lithium-Ion  NomV=3.6  NomQ=4  SOC=30  Batt_Tr=1  PresetModel=on  MaxQ=4  MinV=2.7  FullV=4.1904  Dis_rate=1.7391  R=0.009  Normal_OP=3.6174  expZone="[3.8894     0.19652]"
  Bus Selector : BusSelector  OutputSignals=SOC (%)
  Bus Selector1 : BusSelector  OutputSignals=SOC (%)
  Bus Selector2 : BusSelector  OutputSignals=SOC (%)
  Display : Display
  Display1 : Display
  Display2 : Display
  Ideal Switch : spsIdealSwitchLib/Ideal Switch  Ron=0.001  Lon=0  IC=0  Rs=1e5  Cs=inf  Measurements=off
  Ideal Switch1 : spsIdealSwitchLib/Ideal Switch  Ron=0.001  Lon=0  IC=0  Rs=1e5  Cs=inf  Measurements=off
  Ideal Switch2 : spsIdealSwitchLib/Ideal Switch  Ron=0.001  Lon=0  IC=0  Rs=1e5  Cs=inf  Measurements=off
  MATLAB Function : MATLAB Function  TreatAsAtomicUnit=on
  Scope : Scope
  Scope1 : Scope
  Scope2 : Scope
  Scope3 : Scope  NumInputPorts=3
  Battery - : PMIOPort  Side=Left
  Battery + : PMIOPort  Port=2  Side=Left
  tag scope: EE1=global, EE2=global, EE3=global, socc1=global, socc2=global, socc3=global
  wires:
  Battery2/1 -> Bus Selector1/1
  Bus Selector/1 -> [socc1], Scope/1  "<SOC (%)>"
  [EE3] -> Ideal Switch2/1
  Bus Selector2/1 -> [socc3], Scope2/1  "<SOC (%)>"
  Bus Selector1/1 -> [socc2], Scope1/1  "<SOC (%)>"
  Battery3/1 -> Bus Selector2/1
  [socc2] -> MATLAB Function/2(u2), Display1/1, Scope3/2
  [socc1] -> Display/1, Scope3/1, MATLAB Function/1(u1)
  Battery1/1 -> Bus Selector/1
  [socc3] -> Display2/1, Scope3/3, MATLAB Function/3(u3)
  MATLAB Function/2(s2) -> [EE2]
  MATLAB Function/3(s3) -> [EE3]
  MATLAB Function/1(s1) -> [EE1]
  [EE1] -> Ideal Switch/1
  [EE2] -> Ideal Switch1/1
  connections:
  Ideal Switch1/RConn1 -- Battery1/LConn2
  Ideal Switch/RConn1 -- Battery +/RConn1
  Ideal Switch/LConn1 -- Battery1/LConn1
  Battery -/RConn1 -- Battery3/LConn2
  Ideal Switch2/RConn1 -- Battery2/LConn2
  Ideal Switch2/LConn1 -- Battery3/LConn1
  Ideal Switch1/LConn1 -- Battery2/LConn1

== system aa_IOT/Subsystem5/Subsystem ==
  Battery1 : spsBatteryLib/Battery  BatType=Lithium-Ion  NomV=12  NomQ=100  SOC=100  Batt_Tr=1  PresetModel=on  MaxQ=100  MinV=9  FullV=13.9678  Dis_rate=43.4783  R=0.0012  Normal_OP=90.4348  expZone="[12.9646      4.91304]"
  Battery2 : spsBatteryLib/Battery  BatType=Lithium-Ion  NomV=12  NomQ=100  SOC=60  Batt_Tr=1  PresetModel=on  MaxQ=100  MinV=9  FullV=13.9678  Dis_rate=43.4783  R=0.0012  Normal_OP=90.4348  expZone="[12.9646      4.91304]"
  Battery3 : spsBatteryLib/Battery  BatType=Lithium-Ion  NomV=12  NomQ=100  SOC=30  Batt_Tr=1  PresetModel=on  MaxQ=100  MinV=9  FullV=13.9678  Dis_rate=43.4783  R=0.0012  Normal_OP=90.4348  expZone="[12.9646      4.91304]"
  Bus Selector : BusSelector  OutputSignals=SOC (%),Current (A),Voltage (V)
  Bus Selector1 : BusSelector  OutputSignals=SOC (%),Current (A),Voltage (V)
  Bus Selector2 : BusSelector  OutputSignals=SOC (%),Current (A),Voltage (V)
  Current : Display
  Display : Display
  Display1 : Display
  Display2 : Display
  Ideal Switch : spsIdealSwitchLib/Ideal Switch  Ron=0.001  Lon=0  IC=0  Rs=1e5  Cs=inf  Measurements=off
  Ideal Switch1 : spsIdealSwitchLib/Ideal Switch  Ron=0.001  Lon=0  IC=0  Rs=1e5  Cs=inf  Measurements=off
  Ideal Switch2 : spsIdealSwitchLib/Ideal Switch  Ron=0.001  Lon=0  IC=0  Rs=1e5  Cs=inf  Measurements=off
  MATLAB Function : MATLAB Function  TreatAsAtomicUnit=on
  Scope : Scope
  Scope1 : Scope
  Scope2 : Scope
  Scope3 : Scope  NumInputPorts=3
  Sum : Sum  Inputs=|+++
  Sum1 : Sum  Inputs=|+++
  Voltage : Display
  Battery - : PMIOPort  Side=Left
  Battery + : PMIOPort  Port=2  Side=Left
  tag scope: current_1=global, g1=global, g2=global, g3=global, soc1=global, soc2=global, soc3=global
  wires:
  Battery2/1 -> Bus Selector1/1
  Bus Selector/1 -> Scope/1, [soc1]  "<SOC (%)>"
  [g3] -> Ideal Switch2/1
  Bus Selector2/1 -> Scope2/1, [soc3]  "<SOC (%)>"
  Bus Selector1/1 -> Scope1/1, [soc2]  "<SOC (%)>"
  Battery3/1 -> Bus Selector2/1
  [soc2] -> MATLAB Function/2(u2), Display1/1, Scope3/2
  [soc1] -> Display/1, Scope3/1, MATLAB Function/1(u1)
  Battery1/1 -> Bus Selector/1
  [soc3] -> Display2/1, Scope3/3, MATLAB Function/3(u3)
  MATLAB Function/2(s2) -> [g2]
  MATLAB Function/3(s3) -> [g3]
  MATLAB Function/1(s1) -> [g1]
  [g1] -> Ideal Switch/1
  [g2] -> Ideal Switch1/1
  Bus Selector/2 -> Sum/1  "<Current (A)>"
  Bus Selector1/2 -> Sum/2  "<Current (A)>"
  Bus Selector2/2 -> Sum/3  "<Current (A)>"
  Bus Selector/3 -> [current_1], Current/1, Sum1/1  "<Voltage (V)>"
  Bus Selector1/3 -> Sum1/2  "<Voltage (V)>"
  Bus Selector2/3 -> Sum1/3  "<Voltage (V)>"
  Sum1/1 -> Voltage/1
  connections:
  Ideal Switch2/RConn1 -- Battery2/LConn2
  Battery +/RConn1 -- Ideal Switch/RConn1
  Ideal Switch2/LConn1 -- Battery3/LConn1
  Ideal Switch/LConn1 -- Battery1/LConn1
  Ideal Switch1/RConn1 -- Battery1/LConn2
  Ideal Switch1/LConn1 -- Battery2/LConn1
  Battery -/RConn1 -- Battery3/LConn2

== system aa_IOT/Subsystem6/Subsystem ==
  Battery1 : spsBatteryLib/Battery  BatType=Lithium-Ion  NomV=3.6  NomQ=4  SOC=100  Batt_Tr=1  PresetModel=on  MaxQ=4  MinV=2.7  FullV=4.1904  Dis_rate=1.7391  R=0.009  Normal_OP=3.6174  expZone="[3.8894     0.19652]"
  Battery2 : spsBatteryLib/Battery  BatType=Lithium-Ion  NomV=3.6  NomQ=4  SOC=60  Batt_Tr=1  PresetModel=on  MaxQ=4  MinV=2.7  FullV=4.1904  Dis_rate=1.7391  R=0.009  Normal_OP=3.6174  expZone="[3.8894     0.19652]"
  Battery3 : spsBatteryLib/Battery  BatType=Lithium-Ion  NomV=3.6  NomQ=4  SOC=30  Batt_Tr=1  PresetModel=on  MaxQ=4  MinV=2.7  FullV=4.1904  Dis_rate=1.7391  R=0.009  Normal_OP=3.6174  expZone="[3.8894     0.19652]"
  Bus Selector : BusSelector  OutputSignals=SOC (%)
  Bus Selector1 : BusSelector  OutputSignals=SOC (%)
  Bus Selector2 : BusSelector  OutputSignals=SOC (%)
  Display : Display
  Display1 : Display
  Display2 : Display
  Ideal Switch : spsIdealSwitchLib/Ideal Switch  Ron=0.001  Lon=0  IC=0  Rs=1e5  Cs=inf  Measurements=off
  Ideal Switch1 : spsIdealSwitchLib/Ideal Switch  Ron=0.001  Lon=0  IC=0  Rs=1e5  Cs=inf  Measurements=off
  Ideal Switch2 : spsIdealSwitchLib/Ideal Switch  Ron=0.001  Lon=0  IC=0  Rs=1e5  Cs=inf  Measurements=off
  MATLAB Function : MATLAB Function  TreatAsAtomicUnit=on
  Scope : Scope
  Scope1 : Scope
  Scope2 : Scope
  Scope3 : Scope  NumInputPorts=3
  Battery - : PMIOPort  Side=Left
  Battery + : PMIOPort  Port=2  Side=Left
  tag scope: q1=global, q2=global, q3=global, soc11=global, soc22=global, soc33=global
  wires:
  Battery2/1 -> Bus Selector1/1
  Bus Selector/1 -> [soc11], Scope/1  "<SOC (%)>"
  [q3] -> Ideal Switch2/1
  Bus Selector2/1 -> [soc33], Scope2/1  "<SOC (%)>"
  Bus Selector1/1 -> [soc22], Scope1/1  "<SOC (%)>"
  Battery3/1 -> Bus Selector2/1
  [soc22] -> MATLAB Function/2(u2), Display1/1, Scope3/2
  [soc11] -> Display/1, Scope3/1, MATLAB Function/1(u1)
  Battery1/1 -> Bus Selector/1
  [soc33] -> Display2/1, Scope3/3, MATLAB Function/3(u3)
  MATLAB Function/2(s2) -> [q2]
  MATLAB Function/3(s3) -> [q3]
  MATLAB Function/1(s1) -> [q1]
  [q1] -> Ideal Switch/1
  [q2] -> Ideal Switch1/1
  connections:
  Ideal Switch2/RConn1 -- Battery2/LConn2
  Battery +/RConn1 -- Ideal Switch/RConn1
  Ideal Switch1/LConn1 -- Battery2/LConn1
  Ideal Switch1/RConn1 -- Battery1/LConn2
  Battery -/RConn1 -- Battery3/LConn2
  Ideal Switch2/LConn1 -- Battery3/LConn1
  Ideal Switch/LConn1 -- Battery1/LConn1

== system aa_IOT/Subsystem7/Subsystem ==
  Battery1 : spsBatteryLib/Battery  BatType=Lithium-Ion  NomV=3.6  NomQ=4  SOC=100  Batt_Tr=1  PresetModel=on  MaxQ=4  MinV=2.7  FullV=4.1904  Dis_rate=1.7391  R=0.009  Normal_OP=3.6174  expZone="[3.8894     0.19652]"
  Battery2 : spsBatteryLib/Battery  BatType=Lithium-Ion  NomV=3.6  NomQ=4  SOC=60  Batt_Tr=1  PresetModel=on  MaxQ=4  MinV=2.7  FullV=4.1904  Dis_rate=1.7391  R=0.009  Normal_OP=3.6174  expZone="[3.8894     0.19652]"
  Battery3 : spsBatteryLib/Battery  BatType=Lithium-Ion  NomV=3.6  NomQ=4  SOC=30  Batt_Tr=1  PresetModel=on  MaxQ=4  MinV=2.7  FullV=4.1904  Dis_rate=1.7391  R=0.009  Normal_OP=3.6174  expZone="[3.8894     0.19652]"
  Bus Selector : BusSelector  OutputSignals=SOC (%)
  Bus Selector1 : BusSelector  OutputSignals=SOC (%)
  Bus Selector2 : BusSelector  OutputSignals=SOC (%)
  Display : Display
  Display1 : Display
  Display2 : Display
  Ideal Switch : spsIdealSwitchLib/Ideal Switch  Ron=0.001  Lon=0  IC=0  Rs=1e5  Cs=inf  Measurements=off
  Ideal Switch1 : spsIdealSwitchLib/Ideal Switch  Ron=0.001  Lon=0  IC=0  Rs=1e5  Cs=inf  Measurements=off
  Ideal Switch2 : spsIdealSwitchLib/Ideal Switch  Ron=0.001  Lon=0  IC=0  Rs=1e5  Cs=inf  Measurements=off
  MATLAB Function : MATLAB Function  TreatAsAtomicUnit=on
  Scope : Scope
  Scope1 : Scope
  Scope2 : Scope
  Scope3 : Scope  NumInputPorts=3
  Battery - : PMIOPort  Side=Left
  Battery + : PMIOPort  Port=2  Side=Left
  tag scope: soc111=global, soc222=global, soc333=global, w1=global, w2=global, w3=global
  wires:
  Battery2/1 -> Bus Selector1/1
  Bus Selector/1 -> [soc111], Scope/1  "<SOC (%)>"
  [w3] -> Ideal Switch2/1
  Bus Selector2/1 -> [soc333], Scope2/1  "<SOC (%)>"
  Bus Selector1/1 -> [soc222], Scope1/1  "<SOC (%)>"
  Battery3/1 -> Bus Selector2/1
  [soc222] -> MATLAB Function/2(u2), Display1/1, Scope3/2
  [soc111] -> Display/1, Scope3/1, MATLAB Function/1(u1)
  Battery1/1 -> Bus Selector/1
  [soc333] -> Display2/1, Scope3/3, MATLAB Function/3(u3)
  MATLAB Function/2(s2) -> [w2]
  MATLAB Function/3(s3) -> [w3]
  MATLAB Function/1(s1) -> [w1]
  [w1] -> Ideal Switch/1
  [w2] -> Ideal Switch1/1
  connections:
  Ideal Switch1/RConn1 -- Battery1/LConn2
  Ideal Switch/RConn1 -- Battery +/RConn1
  Ideal Switch/LConn1 -- Battery1/LConn1
  Battery -/RConn1 -- Battery3/LConn2
  Ideal Switch2/RConn1 -- Battery2/LConn2
  Ideal Switch2/LConn1 -- Battery3/LConn1
  Ideal Switch1/LConn1 -- Battery2/LConn1

== system aa_IOT/Vechicle BMS Monitoring/BMS Discharge ==
  Terminal voltage : Inport
  Temperature : Inport  Port=2
  Current : Inport  Port=3
  Constant : Constant  Value=0
  Function logic block : Subsystem
  Switch : Switch  Criteria=u2 ~= 0  SaturateOnIntegerOverflow=off  InputSameDT=off
  Discharge current : Outport
  wires:
  Terminal voltage/1 -> Function logic block/1(Terminal voltage)
  Current/1 -> Switch/3, Function logic block/2(Current)
  Temperature/1 -> Function logic block/3(Temperature)
  Function logic block/1(Discharge Terget) -> Switch/2
  Constant/1 -> Switch/1
  Switch/1 -> Discharge current/1

== system aa_IOT/Vechicle BMS Monitoring1/BMS Discharge ==
  Terminal voltage : Inport
  Temperature : Inport  Port=2
  Current : Inport  Port=3
  Constant : Constant  Value=0
  Function logic block : Subsystem
  Switch : Switch  Criteria=u2 ~= 0  SaturateOnIntegerOverflow=off  InputSameDT=off
  Discharge current : Outport
  wires:
  Terminal voltage/1 -> Function logic block/1(Terminal voltage)
  Current/1 -> Switch/3, Function logic block/2(Current)
  Temperature/1 -> Function logic block/3(Temperature)
  Function logic block/1(Discharge Terget) -> Switch/2
  Constant/1 -> Switch/1
  Switch/1 -> Discharge current/1

== system aa_IOT/Vechicle BMS Monitoring2/BMS Discharge ==
  Terminal voltage : Inport
  Temperature : Inport  Port=2
  Current : Inport  Port=3
  Constant : Constant  Value=0
  Function logic block : Subsystem
  Switch : Switch  Criteria=u2 ~= 0  SaturateOnIntegerOverflow=off  InputSameDT=off
  Discharge current : Outport
  wires:
  Terminal voltage/1 -> Function logic block/1(Terminal voltage)
  Current/1 -> Switch/3, Function logic block/2(Current)
  Temperature/1 -> Function logic block/3(Temperature)
  Function logic block/1(Discharge Terget) -> Switch/2
  Constant/1 -> Switch/1
  Switch/1 -> Discharge current/1

== system aa_IOT/Vechicle BMS Monitoring3/BMS Discharge ==
  Terminal voltage : Inport
  Temperature : Inport  Port=2
  Current : Inport  Port=3
  Constant : Constant  Value=0
  Function logic block : Subsystem
  Switch : Switch  Criteria=u2 ~= 0  SaturateOnIntegerOverflow=off  InputSameDT=off
  Discharge current : Outport
  wires:
  Terminal voltage/1 -> Function logic block/1(Terminal voltage)
  Current/1 -> Switch/3, Function logic block/2(Current)
  Temperature/1 -> Function logic block/3(Temperature)
  Function logic block/1(Discharge Terget) -> Switch/2
  Constant/1 -> Switch/1
  Switch/1 -> Discharge current/1

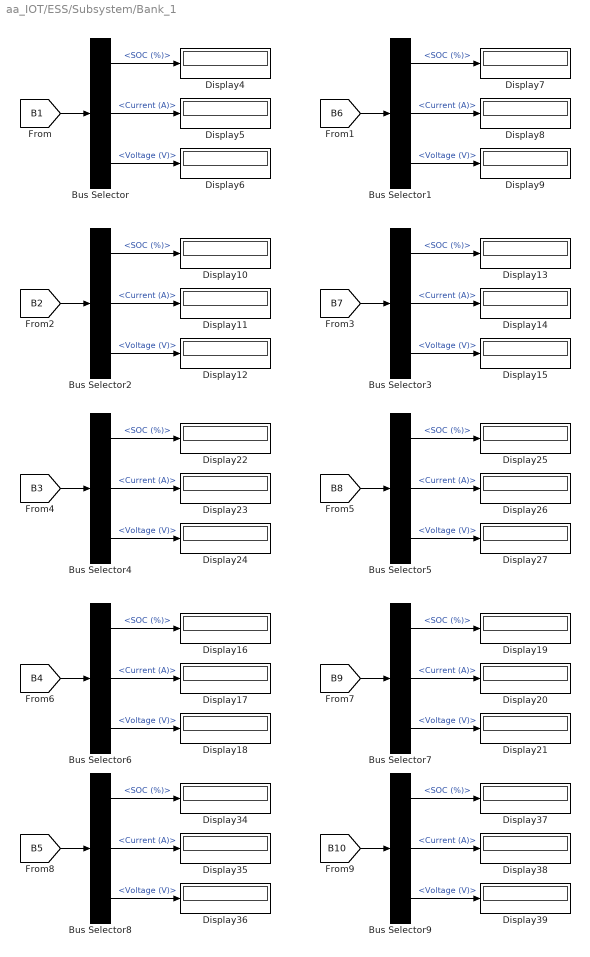
== system aa_IOT/ESS/Subsystem/Bank_1 ==
  Bus Selector{,1..9} (10 alike) : BusSelector  OutputSignals=SOC (%),Current (A),Voltage (V)
  Display{4..27,34..39} (30 alike) : Display
  wires:
  Bus Selector4/2 -> Display23/1  "<Current (A)>"
  [B9] -> Bus Selector7/1
  Bus Selector7/3 -> Display21/1  "<Voltage (V)>"
  Bus Selector1/1 -> Display7/1  "<SOC (%)>"
  [B7] -> Bus Selector3/1
  [B8] -> Bus Selector5/1
  Bus Selector1/2 -> Display8/1  "<Current (A)>"
  Bus Selector/3 -> Display6/1  "<Voltage (V)>"
  Bus Selector4/3 -> Display24/1  "<Voltage (V)>"
  [B4] -> Bus Selector6/1
  Bus Selector6/2 -> Display17/1  "<Current (A)>"
  Bus Selector/2 -> Display5/1  "<Current (A)>"
  [B3] -> Bus Selector4/1
  [B6] -> Bus Selector1/1
  Bus Selector7/2 -> Display20/1  "<Current (A)>"
  Bus Selector6/1 -> Display16/1  "<SOC (%)>"
  Bus Selector9/3 -> Display39/1  "<Voltage (V)>"
  Bus Selector3/2 -> Display14/1  "<Current (A)>"
  Bus Selector5/2 -> Display26/1  "<Current (A)>"
  Bus Selector5/1 -> Display25/1  "<SOC (%)>"
  Bus Selector7/1 -> Display19/1  "<SOC (%)>"
  Bus Selector5/3 -> Display27/1  "<Voltage (V)>"
  Bus Selector4/1 -> Display22/1  "<SOC (%)>"
  Bus Selector9/1 -> Display37/1  "<SOC (%)>"
  Bus Selector2/3 -> Display12/1  "<Voltage (V)>"
  Bus Selector6/3 -> Display18/1  "<Voltage (V)>"
  Bus Selector/1 -> Display4/1  "<SOC (%)>"
  Bus Selector1/3 -> Display9/1  "<Voltage (V)>"
  Bus Selector9/2 -> Display38/1  "<Current (A)>"
  [B10] -> Bus Selector9/1
  Bus Selector8/1 -> Display34/1  "<SOC (%)>"
  Bus Selector8/2 -> Display35/1  "<Current (A)>"
  Bus Selector8/3 -> Display36/1  "<Voltage (V)>"
  [B2] -> Bus Selector2/1
  [B5] -> Bus Selector8/1
  Bus Selector2/2 -> Display11/1  "<Current (A)>"
  Bus Selector3/3 -> Display15/1  "<Voltage (V)>"
  Bus Selector3/1 -> Display13/1  "<SOC (%)>"
  Bus Selector2/1 -> Display10/1  "<SOC (%)>"
  [B1] -> Bus Selector/1

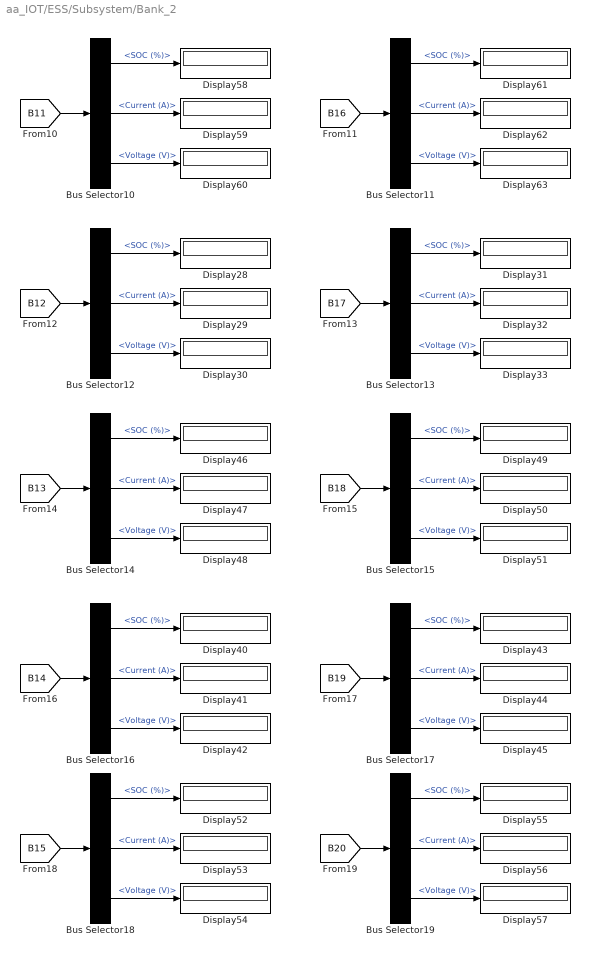
== system aa_IOT/ESS/Subsystem/Bank_2 ==
  Bus Selector{10..19} (10 alike) : BusSelector  OutputSignals=SOC (%),Current (A),Voltage (V)
  Display{28..33,40..63} (30 alike) : Display
  wires:
  Bus Selector17/3 -> Display45/1  "<Voltage (V)>"
  [B16] -> Bus Selector11/1
  Bus Selector16/1 -> Display40/1  "<SOC (%)>"
  Bus Selector12/1 -> Display28/1  "<SOC (%)>"
  [B15] -> Bus Selector18/1
  Bus Selector11/3 -> Display63/1  "<Voltage (V)>"
  [B13] -> Bus Selector14/1
  [B14] -> Bus Selector16/1
  Bus Selector14/3 -> Display48/1  "<Voltage (V)>"
  Bus Selector15/3 -> Display51/1  "<Voltage (V)>"
  [B19] -> Bus Selector17/1
  Bus Selector13/3 -> Display33/1  "<Voltage (V)>"
  Bus Selector19/3 -> Display57/1  "<Voltage (V)>"
  Bus Selector19/1 -> Display55/1  "<SOC (%)>"
  Bus Selector19/2 -> Display56/1  "<Current (A)>"
  Bus Selector16/2 -> Display41/1  "<Current (A)>"
  [B12] -> Bus Selector12/1
  Bus Selector18/1 -> Display52/1  "<SOC (%)>"
  Bus Selector10/2 -> Display59/1  "<Current (A)>"
  Bus Selector14/2 -> Display47/1  "<Current (A)>"
  Bus Selector10/3 -> Display60/1  "<Voltage (V)>"
  Bus Selector18/2 -> Display53/1  "<Current (A)>"
  Bus Selector13/1 -> Display31/1  "<SOC (%)>"
  Bus Selector14/1 -> Display46/1  "<SOC (%)>"
  Bus Selector11/1 -> Display61/1  "<SOC (%)>"
  Bus Selector15/2 -> Display50/1  "<Current (A)>"
  Bus Selector15/1 -> Display49/1  "<SOC (%)>"
  [B11] -> Bus Selector10/1
  Bus Selector17/2 -> Display44/1  "<Current (A)>"
  Bus Selector11/2 -> Display62/1  "<Current (A)>"
  Bus Selector13/2 -> Display32/1  "<Current (A)>"
  Bus Selector12/3 -> Display30/1  "<Voltage (V)>"
  Bus Selector18/3 -> Display54/1  "<Voltage (V)>"
  [B18] -> Bus Selector15/1
  [B17] -> Bus Selector13/1
  Bus Selector10/1 -> Display58/1  "<SOC (%)>"
  Bus Selector12/2 -> Display29/1  "<Current (A)>"
  [B20] -> Bus Selector19/1
  Bus Selector16/3 -> Display42/1  "<Voltage (V)>"
  Bus Selector17/1 -> Display43/1  "<SOC (%)>"
